simulink model "test"  (R2020b)
settings: Solver=VariableStepAuto  StartTime=0.0  StopTime=100.0  RelTol=1e-3
settings Model: Creator=Dogukan  LastModifiedBy=Dogukan

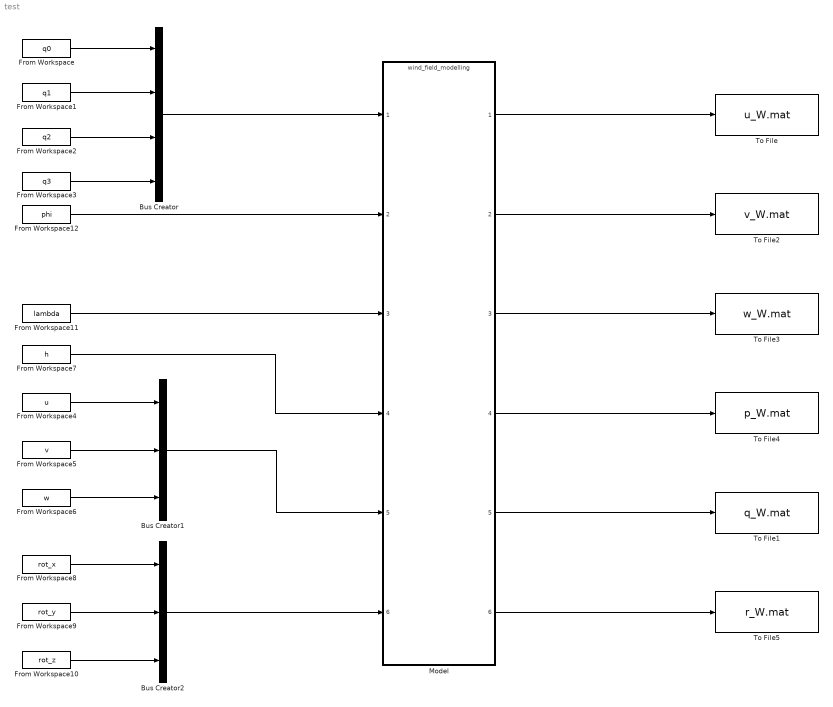
== system test ==
  Bus Creator : BusCreator  Inputs=4
  Bus Creator1 : BusCreator  Inputs=3
  Bus Creator2 : BusCreator  Inputs=3
  From Workspace : FromWorkspace  VariableName=q0
  From Workspace1 : FromWorkspace  VariableName=q1
  From Workspace10 : FromWorkspace  VariableName=rot_z
  From Workspace11 : FromWorkspace  VariableName=lambda
  From Workspace12 : FromWorkspace  VariableName=phi
  From Workspace2 : FromWorkspace  VariableName=q2
  From Workspace3 : FromWorkspace  VariableName=q3
  From Workspace4 : FromWorkspace  VariableName=u
  From Workspace5 : FromWorkspace  VariableName=v
  From Workspace6 : FromWorkspace  VariableName=w
  From Workspace7 : FromWorkspace  VariableName=h
  From Workspace8 : FromWorkspace  VariableName=rot_x
  From Workspace9 : FromWorkspace  VariableName=rot_y
  Model : ModelReference  ModelNameDialog=wind_field_modelling.slx  SimulationMode=Normal  ModelReferenceVersion=1.20
  To File : ToFile  Filename=u_W.mat  MatrixName=u_W  SaveFormat=Timeseries
  To File1 : ToFile  Filename=q_W.mat  MatrixName=q_W  SaveFormat=Timeseries
  To File2 : ToFile  Filename=v_W.mat  MatrixName=v_W  SaveFormat=Timeseries
  To File3 : ToFile  Filename=w_W.mat  MatrixName=w_W  SaveFormat=Timeseries
  To File4 : ToFile  Filename=p_W.mat  MatrixName=p_W  SaveFormat=Timeseries
  To File5 : ToFile  Filename=r_W.mat  MatrixName=r_W  SaveFormat=Timeseries
  wires:
  From Workspace/1 -> Bus Creator/1
  From Workspace1/1 -> Bus Creator/2
  From Workspace2/1 -> Bus Creator/3
  From Workspace3/1 -> Bus Creator/4
  Bus Creator/1 -> Model/1
  From Workspace4/1 -> Bus Creator1/1
  From Workspace5/1 -> Bus Creator1/2
  From Workspace6/1 -> Bus Creator1/3
  Bus Creator1/1 -> Model/5
  From Workspace7/1 -> Model/4
  From Workspace8/1 -> Bus Creator2/1
  From Workspace9/1 -> Bus Creator2/2
  From Workspace10/1 -> Bus Creator2/3
  Bus Creator2/1 -> Model/6
  From Workspace12/1 -> Model/2
  From Workspace11/1 -> Model/3
  Model/1 -> To File/1
  Model/5 -> To File1/1
  Model/2 -> To File2/1
  Model/3 -> To File3/1
  Model/4 -> To File4/1
  Model/6 -> To File5/1
